simulink subsystem "BrakingHydraulicsDiscBrakesRearSSC"  (R2024b)
settings: Solver=VariableStepAuto  StartTime=0.0  StopTime=10.0  RelTol=1e-3
undefined symbols (not defined in the file): AxlRL, AxlRR
libraries: sdl_lib x2, nesl_utility_internal x2
settings Model: ModifiedByFormat=The MathWorks, Inc.  Creator=The MathWorks, Inc.  LastModifiedBy=The MathWorks, Inc.
settings OptimizationCC: ReuseModelBlockBuffer=off
settings RTWCC: GPUComputeCapability=3.5  LargeConstantGeneration=WriteOnlyDNNConstantsToDataFiles

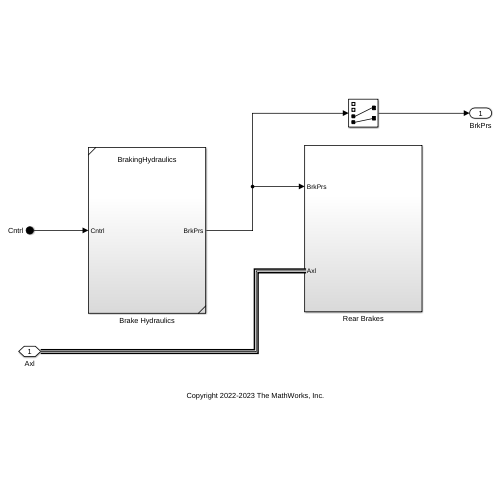
[thumbnail: Simulink's stored preview of the top-level diagram]
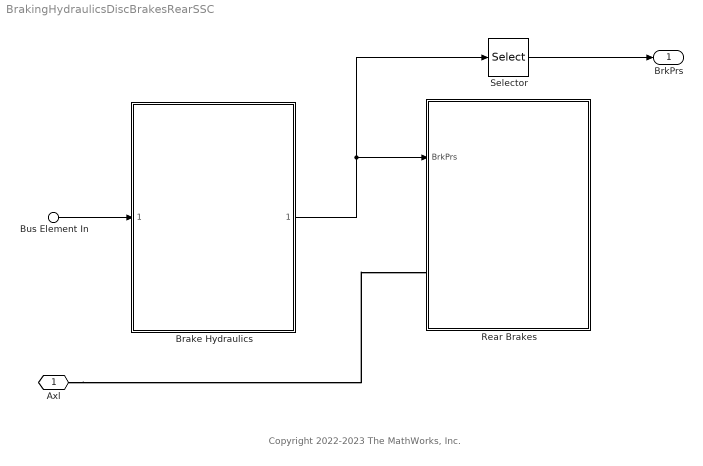
== system BrakingHydraulicsDiscBrakesRearSSC ==
  note: Copyright 2022-2023 The MathWorks, Inc.
  Bus Element In : Inport  PortName=Cntrl
  Brake Hydraulics : Subsystem  ReferencedSubsystem=BrakingHydraulics
  Rear Brakes : Subsystem
  Selector : Selector  InputPortWidth=4  IndexOptions=Index vector (dialog)  Indices=[3 4]  OutputSizes=1
  Axl : PMIOPort  Side=Right
  BrkPrs : Outport
  wires:
  Bus Element In/1 -> Brake Hydraulics/1
  Brake Hydraulics/1 -> Selector/1, Rear Brakes/1(BrkPrs)
  Selector/1 -> BrkPrs/1
  connections:
  Axl/RConn1 -- Rear Brakes/LConn1

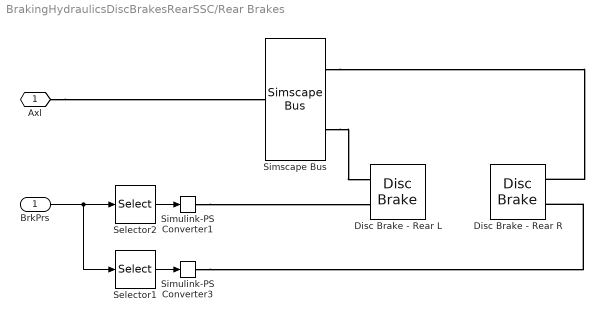
== system BrakingHydraulicsDiscBrakesRearSSC/Rear Brakes ==
  BrkPrs : Inport
  Disc Brake - Rear L : sdl_lib/Brakes & Detents/Rotational/Disc Brake  r_mean=PlntBrkPadMeanRadiusRear m  bore=PlntBrkActrBoreRear m  n_pads=PlntBrkNumPadsRear  thermal_port=simscape.enum.thermaleffects.omit  mu_static=PlntBrkStcFricCffRear  mu_coulomb=PlntBrkKinFricCffRear  temperature_TLU=[280, 300, 320] K  mu_static_TLU=[.9, .8, .7]  mu_coulomb_TLU=[.8, .7, .6]  brkwy_vel=PlntBrkBreakFricVelRear rad/s  visc_coef=PlntBrkViscFricRear N*m*s/rad  thermal_mass=50 kJ/K  temperature_specify=off  temperature_priority=High  temperature=300 K  temperature_nominal_specify=off  temperature_nominal_value=1  temperature_nominal_unit=K
  Disc Brake - Rear R : sdl_lib/Brakes & Detents/Rotational/Disc Brake  r_mean=PlntBrkPadMeanRadiusRear m  bore=PlntBrkActrBoreRear m  n_pads=PlntBrkNumPadsRear  thermal_port=simscape.enum.thermaleffects.omit  mu_static=PlntBrkStcFricCffRear  mu_coulomb=PlntBrkKinFricCffRear  temperature_TLU=[280, 300, 320] K  mu_static_TLU=[.9, .8, .7]  mu_coulomb_TLU=[.8, .7, .6]  brkwy_vel=PlntBrkBreakFricVelRear rad/s  visc_coef=PlntBrkViscFricRear N*m*s/rad  thermal_mass=50 kJ/K  temperature_specify=off  temperature_priority=High  temperature=300 K  temperature_nominal_specify=off  temperature_nominal_value=1  temperature_nominal_unit=K
  Selector1 : Selector  InputPortWidth=4  IndexOptions=Index vector (dialog)  Indices=[4]  OutputSizes=1
  Selector2 : Selector  InputPortWidth=4  IndexOptions=Index vector (dialog)  Indices=[3]  OutputSizes=1
  Simscape Bus : SimscapeBus  HierarchyStrings=AxlRR;AxlRL
  Simulink-PS Converter1 : nesl_utility_internal/Simulink-PS Converter  PhysicalDomain=network_engine_domain  SubClassName=ps_input  LeftPortType=input  RightPortType=output  PseudoPeriodic=off  Frequencies=[]  NoiseDistribution=none  NoiseParameters=[]  Unit=Pa  AffineConversion=off  FilteringAndDerivatives=provide  SimscapeFilterOrder=1  InputFilterTimeConstant=0.001  UdotUserProvided=0
  Simulink-PS Converter3 : nesl_utility_internal/Simulink-PS Converter  PhysicalDomain=network_engine_domain  SubClassName=ps_input  LeftPortType=input  RightPortType=output  PseudoPeriodic=off  Frequencies=[]  NoiseDistribution=none  NoiseParameters=[]  Unit=Pa  AffineConversion=off  FilteringAndDerivatives=provide  SimscapeFilterOrder=1  InputFilterTimeConstant=0.001  UdotUserProvided=0
  Axl : PMIOPort  Side=Left
  wires:
  Selector2/1 -> Simulink-PS Converter1/1
  BrkPrs/1 -> Selector2/1, Selector1/1
  Selector1/1 -> Simulink-PS Converter3/1
  connections:
  Simscape Bus/LConn1 -- Disc Brake - Rear R/LConn2
  Axl/RConn1 -- Simscape Bus/RConn1
  Simulink-PS Converter1/RConn1 -- Disc Brake - Rear L/LConn1
  Simulink-PS Converter3/RConn1 -- Disc Brake - Rear R/LConn1
  Simscape Bus/LConn2 -- Disc Brake - Rear L/LConn2
